simulink model "ReplayFlight_SensorMcu"  (Simulink 7.8)
settings: Solver=FixedStepDiscrete  StartTime=0.0  StopTime=time(end)  FixedStep=.01  RelTol=1e-3
values from neighbouring files (symbols this model uses):
  apSampleTime = 0.01    [Load_Replay.m]    (also in loadReplayMay2013.m; loadTuneRollReplay_May2013.m)
  baseHeight = GS_location(1)    [Load_Replay.m]    (also in loadReplayMay2013.m; loadTuneRollReplay_May2013.m)
  baseTemp = 288.215    [GetBaroAlt.m]
  GS_location = [180 36.9898376464844 -122.051963806152]    [Load_Replay.m]    (also in loadReplayMay2013.m; loadTuneRollReplay_May2013.m)
undefined symbols (not defined in the file or in its folder): barAdjust, baroCutTemp, baroOffset, baroScale, barTGain1, barTGain2, barTMean1, barTMean2, cubeAccelGain16405, cubeGyroGain16405, cubeMagGain16405, DiscIntNeverNeededParam, gaind, getGSLocation, Init_onlyOnce, Init_Reset, lapseRate, lowRateSensorCutoff, magMeanTemp, magOffset, magScale, magTempK, mainSensorCutoff, maxDynPressure, param_mag, pitAdjust, pitCutTemp, pitotOffset, pitotScale, pitTGain1, pitTGain2, pitTMean1, pitTMean2, polesd, powerOffset, powerScale, pressureSensorCutoff, q_quat, T, tempOffset, tempScale, Vb_0, y1, zerosd
libraries: aerolibconvert2 x10, simulink x7, SLUGS_Library x6, aerolibutil x4, dsPICdrivers x2, dspmtrx3 x1
(part 1 of 3)
settings Model: Creator=Administrator  LastModifiedBy=User
settings OptimizationCC: InitFltsAndDblsToZero=on
settings DebuggingCC: SaveWithParameterizedLinksMsg=none  FcnCallInpInsideContextMsg=Use local settings  StrictBusMsg=Warning
settings SFSimCC: SimParseCustomCode=off
settings GRTTargetCC: TargetFcnLib=ansi_tfl_tmw.mat

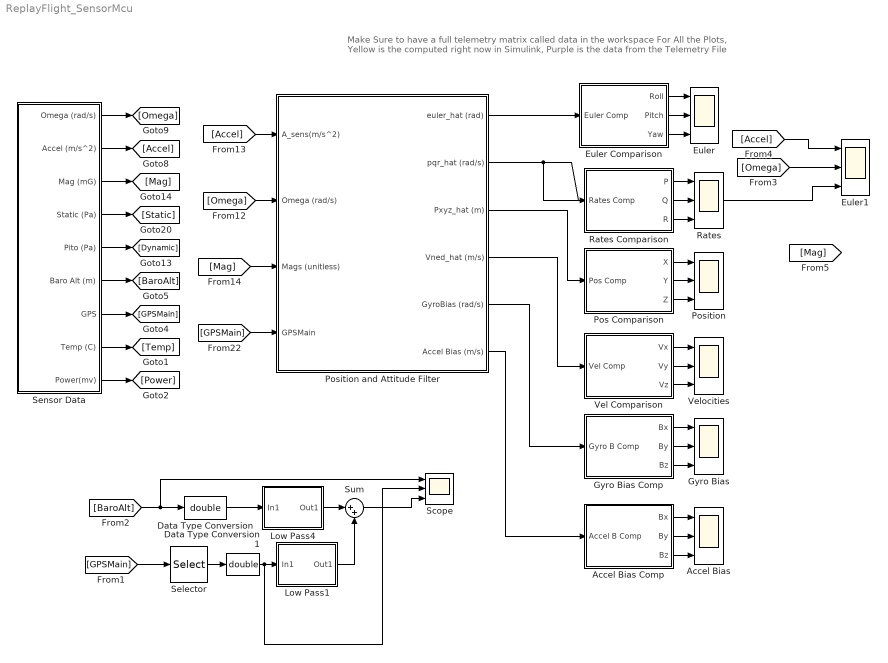
== system ReplayFlight_SensorMcu ==
  note: Make Sure to have a full telemetry matrix
      | called data in the workspace
      |
      | For All the Plots, Yellow is the computed right now in Simulink,
      |  Purple is the data from the Telemetry File
  Accel Bias : Scope  NumInputPorts=3
      settings: YMin=-5~-5~-5  YMax=5~5~5  SaveName=ScopeData5
  Accel Bias Comp : Subsystem
  Data Type Conversion : DataTypeConversion  OutDataTypeStr=double
  Data Type Conversion1 : DataTypeConversion  OutDataTypeStr=double
  Euler : Scope  NumInputPorts=3
      settings: YMin=-5~-5~-5  YMax=5~5~5
  Euler Comparison : Subsystem
  Euler1 : Scope  NumInputPorts=3
      settings: YMin=-5~-5~-5  YMax=5~5~5  SaveName=ScopeData7
  Gyro Bias : Scope  NumInputPorts=3
      settings: YMin=-5~-5~-5  YMax=5~5~5  SaveName=ScopeData4
  Gyro Bias Comp : Subsystem
  Low Pass1 : Subsystem  mask(DiscretizedZeroPole){Zeros=[0], Poles=[-1], Gain=1, AbsTol=auto, SampleTime=T, method=tustin, Wc=1}
      mask prompts: Zeros "Zeros (enter in s-main:)"; Poles "Poles (enter in s-domain:)"; Gain "Gain (enter in s-domain:)"; AbsTol "Absolute tolerance:"; SampleTime "Sample time:"; Wc "Critical Frequency (Hz):"
      mask help: Continuous mask uses c2d to transform parameters onto the Discrete Zero-Pole block inside.
      mask init:
      | st=SampleTime;
      | if length(st)>1
      |     st=SampleTime(1);
      | end
      | if(st>0)
      |     [zerosd,polesd,gaind] = sldiscutil('disczpk', {st,method,Wc,Zeros,Poles,Gain});
      | end	
      | s = get_param(gcb,'maskvalues');
      | zeross = s{1};
      | poless = s{2};
      | gainss = s{3};
      | %zerosc = eval(zeross);
      | %polesc = eval(poless);
      | %gainsc = eval(gainss);
      | sldiscutil('initzpkmask', st);
      | if(st==0)
      | set_param([gcb '/Zero Pole'], 'AbsoluteTolerance', AbsTol);
      | end
      mask StyleString: edit,edit,edit,edit,edit,popup(zoh|foh|tustin|prewarp|matched),edit
      mask CallbackString: |||||hidecrit|
      mask Display:
      | droots(zeross,poless,gainss)
      | text( 0.5, 1.0, method, 'verticalAlignment','top')
  Low Pass4 : Subsystem  mask(DiscretizedZeroPole){Zeros=[], Poles=[-0.3], Gain=0.3, AbsTol=auto, SampleTime=T, method=tustin, Wc=1}
      mask prompts: Zeros "Zeros (enter in s-main:)"; Poles "Poles (enter in s-domain:)"; Gain "Gain (enter in s-domain:)"; AbsTol "Absolute tolerance:"; SampleTime "Sample time:"; Wc "Critical Frequency (Hz):"
      mask help: Continuous mask uses c2d to transform parameters onto the Discrete Zero-Pole block inside.
      mask init: same as ReplayFlight_SensorMcu/Low Pass1
      mask StyleString: edit,edit,edit,edit,edit,popup(zoh|foh|tustin|prewarp|matched),edit
      mask CallbackString: |||||hidecrit|
      mask Display:
      | droots(zeross,poless,gainss)
      | text( 0.5, 1.0, method, 'verticalAlignment','top')
  Pos Comparison : Subsystem
  Position : Scope  NumInputPorts=3
      settings: YMin=-5~-5~-5  YMax=5~5~5  SaveName=ScopeData2
  Position and Attitude Filter : Subsystem
  Rates : Scope  NumInputPorts=3
      settings: YMin=-5~-5~-5  YMax=5~5~5
  Rates Comparison : Subsystem
  Scope : Scope  NumInputPorts=3
      settings: TimeRange=600  YMin=165.625~140~202.34375  YMax=386.875~280~333.59375  SaveName=ScopeData6
  Selector : Selector  InputPortWidth=5  IndexOptions=Index vector (dialog)  Indices=[3]  OutputSizes=1
  Sensor Data : Subsystem
  Sum : Sum  Inputs=|++
  Vel Comparison : Subsystem
  Velocities : Scope  NumInputPorts=3
      settings: YMin=-5~-5~-5  YMax=5~5~5  SaveName=ScopeData3
  wires:
  [Omega] -> Position and Attitude Filter/2(Omega (rad/s))
  [Accel] -> Position and Attitude Filter/1(A_sens(m/s^2))
  [Mag] -> Position and Attitude Filter/3(Mags (unitless))
  [GPSMain] -> Position and Attitude Filter/4(GPSMain)
  Sensor Data/2(Accel (m/s^2)) -> [Accel]
  Sensor Data/1(Omega (rad/s)) -> [Omega]
  Sensor Data/3(Mag (mG)) -> [Mag]
  Sensor Data/4(Static (Pa)) -> [Static]
  Sensor Data/5(Pito (Pa)) -> [Dynamic]
  Sensor Data/6(Baro Alt (m)) -> [BaroAlt]
  Sensor Data/7(GPS) -> [GPSMain]
  Sensor Data/8(Temp (C)) -> [Temp]
  Sensor Data/9(Power(mv)) -> [Power]
  Euler Comparison/1(Roll) -> Euler/1
  Euler Comparison/2(Pitch) -> Euler/2
  Euler Comparison/3(Yaw) -> Euler/3
  Position and Attitude Filter/1(euler_hat (rad)) -> Euler Comparison/1(Euler Comp)
  Rates Comparison/1(P) -> Rates/1
  Rates Comparison/2(Q) -> Rates/2
  Rates Comparison/3(R) -> Rates/3
  Position and Attitude Filter/2(pqr_hat (rad/s)) -> Rates Comparison/1(Rates Comp), Euler1/3
  Pos Comparison/3(Z) -> Position/3
  Position and Attitude Filter/3(Pxyz_hat (m)) -> Pos Comparison/1(Pos Comp)
  Pos Comparison/1(X) -> Position/1
  Pos Comparison/2(Y) -> Position/2
  Vel Comparison/3(Vz) -> Velocities/3
  Vel Comparison/2(Vy) -> Velocities/2
  Vel Comparison/1(Vx) -> Velocities/1
  Position and Attitude Filter/4(Vned_hat (m/s)) -> Vel Comparison/1(Vel Comp)
  Gyro Bias Comp/3(Bz) -> Gyro Bias/3
  Gyro Bias Comp/2(By) -> Gyro Bias/2
  Gyro Bias Comp/1(Bx) -> Gyro Bias/1
  Position and Attitude Filter/5(GyroBias (rad/s)) -> Gyro Bias Comp/1(Gyro B Comp)
  Accel Bias Comp/3(Bz) -> Accel Bias/3
  Accel Bias Comp/1(Bx) -> Accel Bias/1
  Accel Bias Comp/2(By) -> Accel Bias/2
  Position and Attitude Filter/6(Accel Bias (m/s)) -> Accel Bias Comp/1(Accel B Comp)
  [GPSMain] -> Selector/1
  [BaroAlt] -> Data Type Conversion/1, Scope/1
  Selector/1 -> Data Type Conversion1/1
  Low Pass4/1(Out1) -> Sum/1
  Low Pass1/1(Out1) -> Sum/2
  Sum/1 -> Scope/3
  Data Type Conversion/1 -> Low Pass4/1(In1)
  Data Type Conversion1/1 -> Low Pass1/1(In1), Scope/2
  [Omega] -> Euler1/2
  [Accel] -> Euler1/1

== system ReplayFlight_SensorMcu/Accel Bias Comp ==
  Accel B Comp : Inport
  Accel Bias : Subsystem
  Demux : Demux  Outputs=3
  Demux1 : Demux  Outputs=3
  Mux : Mux  Inputs=2
  Mux1 : Mux  Inputs=2
  Mux2 : Mux  Inputs=2
  Bx : Outport
  By : Outport  Port=2
  Bz : Outport  Port=3
  wires:
  Demux1/3 -> Mux2/2
  Demux1/2 -> Mux1/2
  Demux1/1 -> Mux/2
  Accel Bias/1(A bias) -> Demux1/1
  Demux/3 -> Mux2/1
  Demux/2 -> Mux1/1
  Demux/1 -> Mux/1
  Accel B Comp/1 -> Demux/1
  Mux2/1 -> Bz/1
  Mux1/1 -> By/1
  Mux/1 -> Bx/1

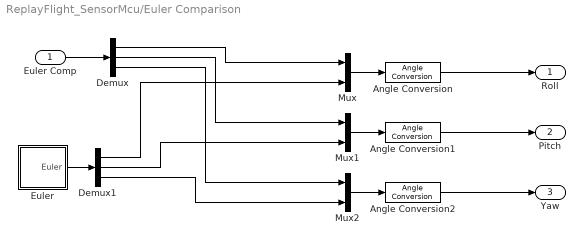
== system ReplayFlight_SensorMcu/Euler Comparison ==
  Euler Comp : Inport
  Angle Conversion : aerolibconvert2/Angle Conversion  IU=rad  OU=deg
  Angle Conversion1 : aerolibconvert2/Angle Conversion  IU=rad  OU=deg
  Angle Conversion2 : aerolibconvert2/Angle Conversion  IU=rad  OU=deg
  Demux : Demux  Outputs=3
  Demux1 : Demux  Outputs=3
  Euler : Subsystem
  Mux : Mux  Inputs=2
  Mux1 : Mux  Inputs=2
  Mux2 : Mux  Inputs=2
  Roll : Outport
  Pitch : Outport  Port=2
  Yaw : Outport  Port=3
  wires:
  Mux/1 -> Angle Conversion/1
  Mux1/1 -> Angle Conversion1/1
  Mux2/1 -> Angle Conversion2/1
  Euler Comp/1 -> Demux/1
  Demux/1 -> Mux/1
  Demux/2 -> Mux1/1
  Demux/3 -> Mux2/1
  Euler/1(Euler) -> Demux1/1
  Demux1/1 -> Mux/2
  Demux1/2 -> Mux1/2
  Demux1/3 -> Mux2/2
  Angle Conversion/1 -> Roll/1
  Angle Conversion1/1 -> Pitch/1
  Angle Conversion2/1 -> Yaw/1

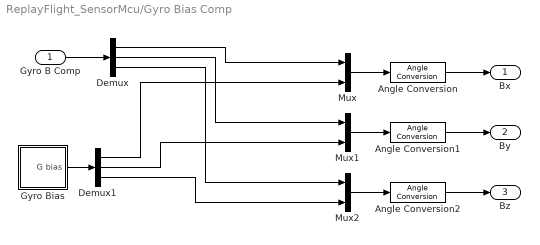
== system ReplayFlight_SensorMcu/Gyro Bias Comp ==
  Gyro B Comp : Inport
  Angle Conversion : aerolibconvert2/Angle Conversion  IU=rad  OU=deg
  Angle Conversion1 : aerolibconvert2/Angle Conversion  IU=rad  OU=deg
  Angle Conversion2 : aerolibconvert2/Angle Conversion  IU=rad  OU=deg
  Demux : Demux  Outputs=3
  Demux1 : Demux  Outputs=3
  Gyro Bias : Subsystem
  Mux : Mux  Inputs=2
  Mux1 : Mux  Inputs=2
  Mux2 : Mux  Inputs=2
  Bx : Outport
  By : Outport  Port=2
  Bz : Outport  Port=3
  wires:
  Mux/1 -> Angle Conversion/1
  Mux1/1 -> Angle Conversion1/1
  Mux2/1 -> Angle Conversion2/1
  Gyro B Comp/1 -> Demux/1
  Demux/1 -> Mux/1
  Demux/2 -> Mux1/1
  Demux/3 -> Mux2/1
  Gyro Bias/1(G bias) -> Demux1/1
  Demux1/1 -> Mux/2
  Demux1/2 -> Mux1/2
  Demux1/3 -> Mux2/2
  Angle Conversion/1 -> Bx/1
  Angle Conversion1/1 -> By/1
  Angle Conversion2/1 -> Bz/1

== system ReplayFlight_SensorMcu/Low Pass1 ==
  In1 : Inport
  Discrete Zero-Pole : DiscreteZeroPole  Zeros=zerosd  Poles=polesd  Gain=gaind  SampleTime=SampleTime
  Out1 : Outport
  wires:
  Discrete Zero-Pole/1 -> Out1/1
  In1/1 -> Discrete Zero-Pole/1

== system ReplayFlight_SensorMcu/Low Pass4 ==
  In1 : Inport
  Discrete Zero-Pole : DiscreteZeroPole  Zeros=zerosd  Poles=polesd  Gain=gaind  SampleTime=SampleTime
  Out1 : Outport
  wires:
  In1/1 -> Discrete Zero-Pole/1
  Discrete Zero-Pole/1 -> Out1/1

== system ReplayFlight_SensorMcu/Pos Comparison ==
  Pos Comp : Inport
  Demux : Demux  Outputs=3
  Demux1 : Demux  Outputs=3
  Mux : Mux  Inputs=2
  Mux1 : Mux  Inputs=2
  Mux2 : Mux  Inputs=2
  Pos : Subsystem
  X : Outport
  Y : Outport  Port=2
  Z : Outport  Port=3
  wires:
  Mux/1 -> X/1
  Mux1/1 -> Y/1
  Mux2/1 -> Z/1
  Pos Comp/1 -> Demux/1
  Demux/1 -> Mux/1
  Demux/2 -> Mux1/1
  Demux/3 -> Mux2/1
  ? -> Demux1/1
  Demux1/1 -> Mux/2
  Demux1/2 -> Mux1/2
  Demux1/3 -> Mux2/2

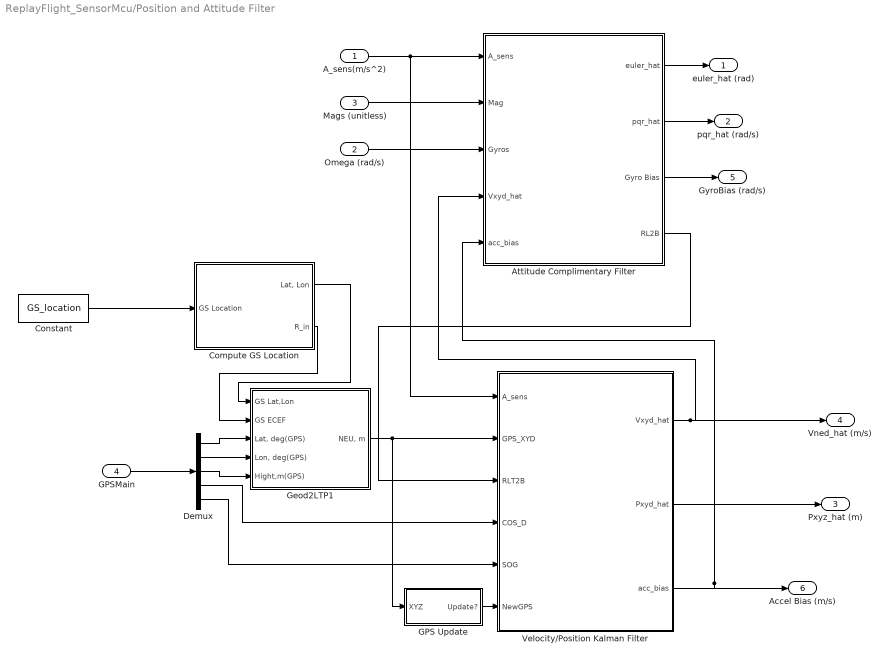
== system ReplayFlight_SensorMcu/Position and Attitude Filter ==
  A_sens(m/s^2) : Inport
  Omega (rad/s) : Inport  Port=2
  Mags (unitless) : Inport  Port=3
  GPSMain : Inport  Port=4
  Attitude Complimentary Filter : Subsystem
  Compute GS Location : Subsystem
  Constant : Constant  Value=GS_location  OutDataTypeStr=single
  Demux : Demux  Outputs=5
  GPS Update : Subsystem  mask{T=0.01}
      mask prompts: T "Sample Time"
  Geod2LTP1 : Subsystem
      mask Description:
      | This block provides transformation of the Geodetic coordinates
      | to the LTP coorinate system. The block uses two consecutive transformations
      | (Geodetic -> ECEF ->LTP).
      | Geodetic coordinates of the LTP origin should also be predetermined.
      mask Help: Oops!
      mask Display: plot(0,0,100,100,[45,40,35,40,40],[85,95,85,95,40],[85,95,85,95,40],[35,40,45,40,40],[60,40,10,20,10,14],[70,40,10,13,10,20],[56,45],[70,70],[60,60],[50,60],[60,60],[30,40],[50,60],[20,20],[30,40],[20,20],[45,55],[35,25],[75,65],[35,25])
  Velocity/Position Kalman Filter : MATLAB Function  TreatAsAtomicUnit=on
  euler_hat (rad) : Outport
  pqr_hat (rad/s) : Outport  Port=2
  Pxyz_hat (m) : Outport  Port=3
  Vned_hat (m/s) : Outport  Port=4
  GyroBias (rad/s) : Outport  Port=5
  Accel Bias (m/s) : Outport  Port=6
  wires:
  Omega (rad/s)/1 -> Attitude Complimentary Filter/3(Gyros)
  Mags (unitless)/1 -> Attitude Complimentary Filter/2(Mag)
  A_sens(m/s^2)/1 -> Attitude Complimentary Filter/1(A_sens), Velocity/Position Kalman Filter/1(A_sens)
  GPS Update/1(Update?) -> Velocity/Position Kalman Filter/6(NewGPS)
  Compute GS Location/1("Lat, Lon") -> Geod2LTP1/1(GS Lat,Lon)
  Compute GS Location/2(R_in) -> Geod2LTP1/2(GS ECEF)
  Demux/3 -> Geod2LTP1/5(Hight,m(GPS))
  Demux/2 -> Geod2LTP1/4("Lon, deg(GPS)")
  Demux/1 -> Geod2LTP1/3("Lat, deg(GPS)")
  Constant/1 -> Compute GS Location/1(GS Location)
  Demux/5 -> Velocity/Position Kalman Filter/5(SOG)
  Demux/4 -> Velocity/Position Kalman Filter/4(COS_D)
  GPSMain/1 -> Demux/1
  Attitude Complimentary Filter/3(Gyro Bias) -> GyroBias (rad/s)/1
  Attitude Complimentary Filter/2(pqr_hat) -> pqr_hat (rad/s)/1
  Attitude Complimentary Filter/1(euler_hat) -> euler_hat (rad)/1
  Attitude Complimentary Filter/4(RL2B) -> Velocity/Position Kalman Filter/3(RLT2B)
  Geod2LTP1/1("NEU, m") -> Velocity/Position Kalman Filter/2(GPS_XYD), GPS Update/1(XYZ)
  Velocity/Position Kalman Filter/3(acc_bias) -> Accel Bias (m/s)/1, Attitude Complimentary Filter/5(acc_bias)
  Velocity/Position Kalman Filter/2(Pxyd_hat) -> Pxyz_hat (m)/1
  Velocity/Position Kalman Filter/1(Vxyd_hat) -> Vned_hat (m/s)/1, Attitude Complimentary Filter/4(Vxyd_hat)

== system ReplayFlight_SensorMcu/Rates Comparison ==
  Rates Comp : Inport
  Angle Conversion : aerolibconvert2/Angle Conversion  IU=rad  OU=deg
  Angle Conversion1 : aerolibconvert2/Angle Conversion  IU=rad  OU=deg
  Angle Conversion2 : aerolibconvert2/Angle Conversion  IU=rad  OU=deg
  Demux : Demux  Outputs=3
  Demux1 : Demux  Outputs=3
  Mux : Mux  Inputs=2
  Mux1 : Mux  Inputs=2
  Mux2 : Mux  Inputs=2
  Rates : Subsystem
  P : Outport
  Q : Outport  Port=2
  R : Outport  Port=3
  wires:
  Angle Conversion2/1 -> R/1
  Angle Conversion1/1 -> Q/1
  Angle Conversion/1 -> P/1
  Demux1/3 -> Mux2/2
  Demux1/2 -> Mux1/2
  Demux1/1 -> Mux/2
  Rates/1(Rates) -> Demux1/1
  Demux/3 -> Mux2/1
  Demux/2 -> Mux1/1
  Demux/1 -> Mux/1
  Rates Comp/1 -> Demux/1
  Mux2/1 -> Angle Conversion2/1
  Mux1/1 -> Angle Conversion1/1
  Mux/1 -> Angle Conversion/1

== system ReplayFlight_SensorMcu/Sensor Data ==
  Sensor Suite : Subsystem
  Omega (rad/s) : Outport
  Accel (m/s^2) : Outport  Port=2
  Mag (mG) : Outport  Port=3
  Static (Pa) : Outport  Port=4
  Pito (Pa) : Outport  Port=5
  Baro Alt (m) : Outport  Port=6
  GPS : Outport  Port=7
  Temp (C) : Outport  Port=8
  Power(mv) : Outport  Port=9
  wires:
  Sensor Suite/7(GPS) -> GPS/1
  Sensor Suite/6(Baro Alt (m)) -> Baro Alt (m)/1
  Sensor Suite/5(Pitot (Pa)) -> Pito (Pa)/1
  Sensor Suite/4(Static (Pa)) -> Static (Pa)/1
  Sensor Suite/3(Mag (normalized)) -> Mag (mG)/1
  Sensor Suite/2(Accel (m/s^2)) -> Accel (m/s^2)/1
  Sensor Suite/1(Omega (rad/s)) -> Omega (rad/s)/1
  Sensor Suite/8(Temp(C)) -> Temp (C)/1
  Sensor Suite/9(Power) -> Power(mv)/1

== system ReplayFlight_SensorMcu/Vel Comparison ==
  Vel Comp : Inport
  Demux : Demux  Outputs=3
  Demux1 : Demux  Outputs=3
  Mux : Mux  Inputs=2
  Mux1 : Mux  Inputs=2
  Mux2 : Mux  Inputs=2
  Vel : Subsystem
  Vx : Outport
  Vy : Outport  Port=2
  Vz : Outport  Port=3
  wires:
  Demux1/3 -> Mux2/2
  Demux1/2 -> Mux1/2
  Demux1/1 -> Mux/2
  ? -> Demux1/1
  Demux/3 -> Mux2/1
  Demux/2 -> Mux1/1
  Demux/1 -> Mux/1
  Vel Comp/1 -> Demux/1
  Mux2/1 -> Vz/1
  Mux1/1 -> Vy/1
  Mux/1 -> Vx/1

== system ReplayFlight_SensorMcu/Accel Bias Comp/Accel Bias ==
  Data Type Conversion3 : DataTypeConversion  OutDataTypeStr=single
  Mux : Mux  Inputs=3
  p : FromWorkspace  VariableName=[time ABI_comp(:,1)]  SampleTime=0.01  OutputAfterFinalValue=Setting to zero
  p1 : FromWorkspace  VariableName=[time ABI_comp(:,2)]  SampleTime=0.01  OutputAfterFinalValue=Setting to zero
  p2 : FromWorkspace  VariableName=[time ABI_comp(:,3)]  SampleTime=0.01  OutputAfterFinalValue=Setting to zero
  A bias : Outport
  wires:
  Data Type Conversion3/1 -> A bias/1
  Mux/1 -> Data Type Conversion3/1
  p2/1 -> Mux/3
  p1/1 -> Mux/2
  p/1 -> Mux/1

== system ReplayFlight_SensorMcu/Euler Comparison/Euler ==
  Data Type Conversion3 : DataTypeConversion  OutDataTypeStr=single
  Mux : Mux  Inputs=3
  p : FromWorkspace  VariableName=[time EUL_comp(:,1)]  SampleTime=0.01  OutputAfterFinalValue=Setting to zero
  p1 : FromWorkspace  VariableName=[time EUL_comp(:,2)]  SampleTime=0.01  OutputAfterFinalValue=Setting to zero
  p2 : FromWorkspace  VariableName=[time EUL_comp(:,3)]  SampleTime=0.01  OutputAfterFinalValue=Setting to zero
  Euler : Outport
  wires:
  p/1 -> Mux/1
  p1/1 -> Mux/2
  p2/1 -> Mux/3
  Mux/1 -> Data Type Conversion3/1
  Data Type Conversion3/1 -> Euler/1

== system ReplayFlight_SensorMcu/Gyro Bias Comp/Gyro Bias ==
  Data Type Conversion3 : DataTypeConversion  OutDataTypeStr=single
  Mux : Mux  Inputs=3
  p : FromWorkspace  VariableName=[time GBI_comp(:,1)]  SampleTime=0.01  OutputAfterFinalValue=Setting to zero
  p1 : FromWorkspace  VariableName=[time GBI_comp(:,2)]  SampleTime=0.01  OutputAfterFinalValue=Setting to zero
  p2 : FromWorkspace  VariableName=[time GBI_comp(:,3)]  SampleTime=0.01  OutputAfterFinalValue=Setting to zero
  G bias : Outport
  wires:
  p/1 -> Mux/1
  p1/1 -> Mux/2
  p2/1 -> Mux/3
  Mux/1 -> Data Type Conversion3/1
  Data Type Conversion3/1 -> G bias/1

== system ReplayFlight_SensorMcu/Pos Comparison/Pos ==
  Data Type Conversion3 : DataTypeConversion  OutDataTypeStr=single
  Mux : Mux  Inputs=3
  p : FromWorkspace  VariableName=[time POS_comp(:,1)]  SampleTime=0.01  OutputAfterFinalValue=Setting to zero
  p1 : FromWorkspace  VariableName=[time POS_comp(:,2)]  SampleTime=0.01  OutputAfterFinalValue=Setting to zero
  p2 : FromWorkspace  VariableName=[time POS_comp(:,3)]  SampleTime=0.01  OutputAfterFinalValue=Setting to zero
  Position : Outport
  wires:
  p/1 -> Mux/1
  p1/1 -> Mux/2
  p2/1 -> Mux/3
  Mux/1 -> Data Type Conversion3/1
  Data Type Conversion3/1 -> Position/1

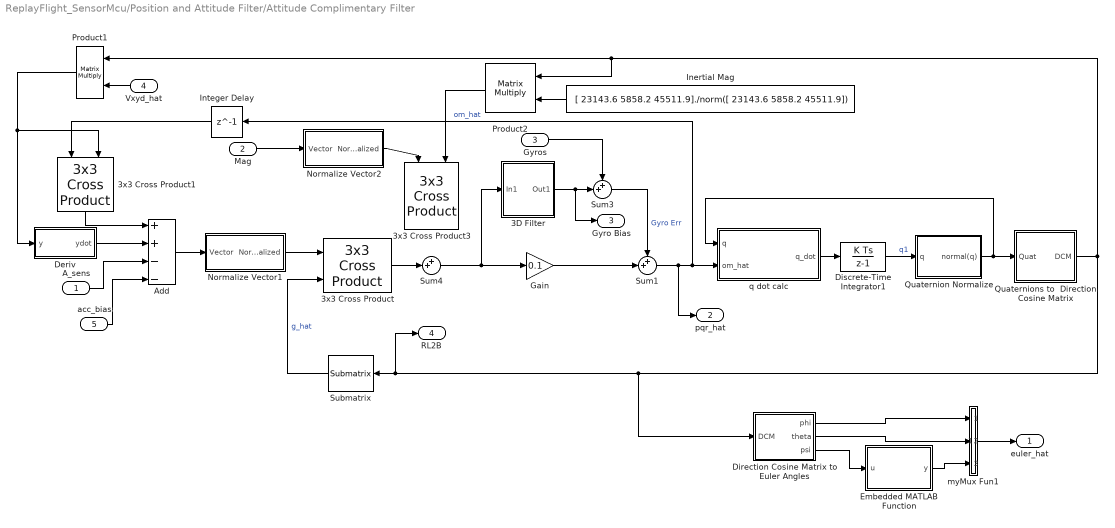
== system ReplayFlight_SensorMcu/Position and Attitude Filter/Attitude Complimentary Filter ==
  A_sens : Inport  PortDimensions=3
  Mag : Inport  Port=2  PortDimensions=3
  Gyros : Inport  Port=3  PortDimensions=3
  Vxyd_hat : Inport  Port=4  PortDimensions=3
  acc_bias : Inport  Port=5  PortDimensions=3
  3D Filter : Subsystem  AncestorBlock=SLUGS_Library/Singnal Routing & Conditioning/3D Filter  RTWFcnName=TustinFilter3D  mask{zval=[], pval=[0], kval=.003, TSample=0.01}
      mask prompts: zval "Zeros"; pval "Poles"; kval "Gains"; TSample "Sample Time"
      settings: RTWFcnNameOpts=User specified  RTWFileNameOpts=Use function name
      mask Display:
      | droots(zval,pval,kval)
      | port_label('input',1,'3D')
  3x3 Cross Product : aerolibutil/3x3 Cross Product
  3x3 Cross Product1 : aerolibutil/3x3 Cross Product
  3x3 Cross Product3 : aerolibutil/3x3 Cross Product
  Add : Sum  Inputs=++--
  "Deriv " : Subsystem
  Direction Cosine Matrix to Euler Angles : Subsystem  AncestorBlock=aerolibtransform2/Direction Cosine Matrix to Euler Angles  mask(DCM2Euler){}
      mask help: Determine an euler orientation (roll, pitch, yaw) from the 3-by-3 direction cosine matrix (DCM). The input DCM transforms vectors from geodetic earth or north-down-east (NED) axes to body axes.
      mask init:
      | aeroicon('aeroblk');
      mask Help: web(asbhelp('directioncosinematrixtoeulerangles'));
      mask Display:
      | port_label('output',1,'\phi','texmode','on')
      | port_label('output',2,'\theta','texmode','on')
      | port_label('output',3,'\psi','texmode','on')
      | port_label('input',1,'DCM_{be}','texmode','on')
  Discrete-Time Integrator1 : DiscreteIntegrator  InitialCondition=q_quat  SampleTime=apSampleTime  LimitOutput=on  UpperSaturationLimit=[1 1 1 1]  LowerSaturationLimit=[-1 -1 -1 -1]  ICPrevOutput=DiscIntNeverNeededParam  ICPrevScaledInput=DiscIntNeverNeededParam
  Embedded MATLAB Function : MATLAB Function  TreatAsAtomicUnit=on
  Gain : Gain  Gain=0.1
  Inertial Mag : Constant  Value="[ 23143.6   5858.2    45511.9]./norm([ 23143.6   5858.2    45511.9])"  OutDataTypeStr=single
  Integer Delay : Delay  DelayLength=1  InputProcessing=Inherited
  Normalize Vector1 : Subsystem  AncestorBlock=SLUGS_Library/Navigation/Normalize Vector
  Normalize Vector2 : Subsystem  AncestorBlock=SLUGS_Library/Navigation/Normalize Vector
  Product1 : Product  Multiplication=Matrix(*)  RndMeth=Zero
  Product2 : Product  Multiplication=Matrix(*)  RndMeth=Zero
  Quaternion Normalize : Subsystem  AncestorBlock=aerolibutil/Quaternion Normalize  mask(Quaternion Normalize){}
      mask help: Normalize a quaternion.
      mask init:
      | aeroicon('aeroblk');
      mask Help: web(asbhelp);
  Quaternions to  Direction Cosine Matrix : Subsystem  AncestorBlock="aerolibtransform2/Quaternions to  Direction Cosine Matrix"  mask(Quaternion2DCM){}
      mask help: Determine the 3-by-3 direction cosine matrix (DCM) from a 4-by-1 quaternion orientation vector. The output DCM transforms vectors from geodetic earth or north-east-down (NED) axes to body axes.
      mask init:
      | aeroicon('aeroblk');
      mask Help: web(asbhelp('quaternionstodirectioncosinematrix'));
      mask Display:
      | port_label('input',1,'q_n_o_r_m','texmode','on')
      | port_label('output',1,'DCM_{be}','texmode','on')
  Submatrix : dspmtrx3/Submatrix  RowSpan=Range of rows  RowStartMode=First  RowStartIndex=1  RowEndMode=Last  RowEndIndex=1  ColSpan=One column  ColStartMode=Last  ColStartIndex=1  ColEndMode=Last  ColEndIndex=1
  Sum1 : Sum  Inputs=++|
  Sum3 : Sum  Inputs=++|
  Sum4 : Sum  Inputs=++|
  myMux Fun1 : MATLAB Function  TreatAsAtomicUnit=on
  q dot calc : MATLAB Function  TreatAsAtomicUnit=on
  euler_hat : Outport
  pqr_hat : Outport  Port=2
  Gyro Bias : Outport  Port=3
  RL2B : Outport  Port=4
  wires:
  Normalize Vector2/1(Normalized) -> 3x3 Cross Product3/1
  Sum3/1 -> Sum1/1  "Gyro Err"
  Gain/1 -> Sum1/2
  Gyros/1 -> Sum3/1
  3D Filter/1(Out1) -> Sum3/2, Gyro Bias/1
  Embedded MATLAB Function/1(y) -> myMux Fun1/3(u3)
  Direction Cosine Matrix to Euler Angles/2(theta) -> myMux Fun1/2(u2)
  Direction Cosine Matrix to Euler Angles/1(phi) -> myMux Fun1/1(u1)
  myMux Fun1/1(y) -> euler_hat/1
  Direction Cosine Matrix to Euler Angles/3(psi) -> Embedded MATLAB Function/1(u)
  Vxyd_hat/1 -> Product1/2
  Product1/1 -> "Deriv "/1(y), 3x3 Cross Product1/2
  Mag/1 -> Normalize Vector2/1(Vector)
  acc_bias/1 -> Add/4
  Add/1 -> Normalize Vector1/1(Vector)
  "Deriv "/1(ydot) -> Add/2
  Quaternion Normalize/1(normal(q)) -> q dot calc/1(q), Quaternions to  Direction Cosine Matrix/1(Quat)
  Discrete-Time Integrator1/1 -> Quaternion Normalize/1(q)  "q1"
  Integer Delay/1 -> 3x3 Cross Product1/1
  Inertial Mag/1 -> Product2/2
  Quaternions to  Direction Cosine Matrix/1(DCM) -> Direction Cosine Matrix to Euler Angles/1(DCM), RL2B/1, Submatrix/1, Product1/1, Product2/1
  Product2/1 -> 3x3 Cross Product3/2
  3x3 Cross Product/1 -> Sum4/2
  Normalize Vector1/1(Normalized) -> 3x3 Cross Product/1
  A_sens/1 -> Add/3
  3x3 Cross Product1/1 -> Add/1
  Sum4/1 -> 3D Filter/1(In1), Gain/1
  Submatrix/1 -> 3x3 Cross Product/2  "g_hat"
  q dot calc/1(q_dot) -> Discrete-Time Integrator1/1
  Sum1/1 -> pqr_hat/1, Integer Delay/1, q dot calc/2(om_hat)  "om_hat"

== system ReplayFlight_SensorMcu/Position and Attitude Filter/Compute GS Location ==
  GS Location : Inport
  Demux : Demux  Outputs=3
  Geod2ECEF1 : Subsystem  mask{Re=6378137, Rp=6356752.3142}
      mask prompts: Re "Enter equatorial radius, m"; Rp "Enter polar radius,m"
  Mux1 : Mux  Inputs=2
  Mux2 : Mux  Inputs=3
  "Lat, Lon" : Outport
  R_in : Outport  Port=2
  wires:
  Mux2/1 -> R_in/1  "R_in"
  Mux1/1 -> "Lat, Lon"/1
  GS Location/1 -> Demux/1
  Demux/3 -> Geod2ECEF1/3(lon,deg), Mux1/1
  Demux/2 -> Geod2ECEF1/2("lat, deg"), Mux1/2
  Demux/1 -> Geod2ECEF1/1("height, m")
  Geod2ECEF1/2("Ye, m ") -> Mux2/2
  Geod2ECEF1/1("Xe, m ") -> Mux2/1
  Geod2ECEF1/3("Ze, m ") -> Mux2/3

== system ReplayFlight_SensorMcu/Position and Attitude Filter/GPS Update ==
  XYZ : Inport
  Data Type Conversion2 : DataTypeConversion  OutDataTypeStr=uint8
  Demux : Demux  Outputs=3
  Detect Change : Subsystem
  Detect Change1 : Subsystem
  Detect Change2 : Subsystem
  Rate Transition : RateTransition  OutPortSampleTime=T
  Saturation1 : Saturate  UpperLimit=1  LowerLimit=0  SampleTime=T
  Sum : Sum  Inputs=3
  Update? : Outport
  wires:
  Data Type Conversion2/1 -> Update?/1
  Rate Transition/1 -> Demux/1
  Saturation1/1 -> Data Type Conversion2/1
  XYZ/1 -> Rate Transition/1
  Sum/1 -> Saturation1/1
  Detect Change2/1(change?) -> Sum/3
  Detect Change1/1(change?) -> Sum/2
  Detect Change/1(change?) -> Sum/1
  Demux/3 -> Detect Change2/1(Data)
  Demux/2 -> Detect Change1/1(Data)
  Demux/1 -> Detect Change/1(Data)

== system ReplayFlight_SensorMcu/Position and Attitude Filter/Geod2LTP1 ==
  GS Lat,Lon : Inport
  GS ECEF : Inport  Port=2
  "Lat, deg(GPS)" : Inport  Port=3
  "Lon, deg(GPS)" : Inport  Port=4
  Hight,m(GPS) : Inport  Port=5
  ECEF2LTP (UEN) : Subsystem
      mask Display: plot(0,0,100,100,[45,40,35,40,40],[85,95,85,95,40],[85,95,85,95,40],[35,40,45,40,40],[60,40,10,20,10,14],[70,40,10,13,10,20],[56,45],[70,70],[60,60],[50,60],[60,60],[30,40],[50,60],[20,20],[30,40],[20,20],[45,55],[35,25],[75,65],[35,25])
  Geod2ECEF1 : Subsystem  mask{Re=6378137, Rp=6356752.3142}
      mask prompts: Re "Enter equatorial radius, m"; Rp "Enter polar radius,m"
  Mux : Mux  Inputs=3
  Reshape : Reshape  OutputDimensionality=Column vector (2-D)
  Reshape1 : Reshape
  Sum1 : Sum  Inputs=|+-  OutDataTypeStr=single  SaturateOnIntegerOverflow=on
  UEN 2 NEU : Gain  Gain=[0 0 1;0 1 0;1 0 0]  Multiplication=Matrix(K*u)  OutDataTypeStr=float('single')  SaturateOnIntegerOverflow=on  ParamDataTypeStr=Inherit: Same as input
  "NEU, m" : Outport
  wires:
  UEN 2 NEU/1 -> Reshape1/1
  Geod2ECEF1/3("Ze, m ") -> Mux/3
  Geod2ECEF1/1("Xe, m ") -> Mux/1
  Geod2ECEF1/2("Ye, m ") -> Mux/2
  "Lat, deg(GPS)"/1 -> Geod2ECEF1/2("lat, deg")
  "Lon, deg(GPS)"/1 -> Geod2ECEF1/3(lon,deg)
  GS Lat,Lon/1 -> ECEF2LTP (UEN)/2("Long, Lat")
  GS ECEF/1 -> Sum1/2
  ECEF2LTP (UEN)/1(Out) -> Reshape/1  "Moving Side"
  Hight,m(GPS)/1 -> Geod2ECEF1/1("height, m")
  Mux/1 -> Sum1/1  "r_mov"
  Sum1/1 -> ECEF2LTP (UEN)/1(ECEF coordinates)
  Reshape/1 -> UEN 2 NEU/1
  Reshape1/1 -> "NEU, m"/1

== system ReplayFlight_SensorMcu/Rates Comparison/Rates ==
  Data Type Conversion3 : DataTypeConversion  OutDataTypeStr=single
  Mux : Mux  Inputs=3
  p : FromWorkspace  VariableName=[time PQR_comp(:,1)]  SampleTime=0.01  OutputAfterFinalValue=Setting to zero
  p1 : FromWorkspace  VariableName=[time PQR_comp(:,2)]  SampleTime=0.01  OutputAfterFinalValue=Setting to zero
  p2 : FromWorkspace  VariableName=[time PQR_comp(:,3)]  SampleTime=0.01  OutputAfterFinalValue=Setting to zero
  Rates : Outport
  wires:
  Data Type Conversion3/1 -> Rates/1
  Mux/1 -> Data Type Conversion3/1
  p2/1 -> Mux/3
  p1/1 -> Mux/2
  p/1 -> Mux/1

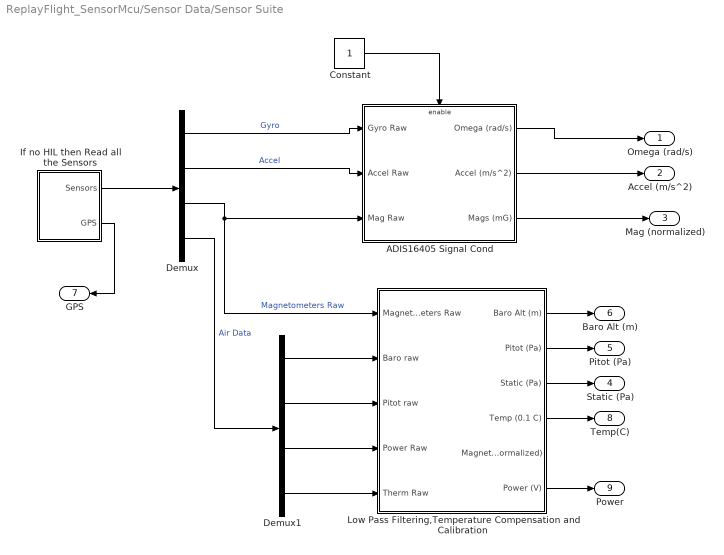
== system ReplayFlight_SensorMcu/Sensor Data/Sensor Suite ==
  "ADIS16405 Signal Cond " : Subsystem
  Constant : Constant
  Demux : Demux  Outputs=[3 3 3 4]
  Demux1 : Demux
  If no HIL then Read all the Sensors : Subsystem
  Low Pass Filtering,Temperature Compensation and Calibration : Subsystem
  Omega (rad/s) : Outport
  Accel (m/s^2) : Outport  Port=2
  Mag (normalized) : Outport  Port=3
  Static (Pa) : Outport  Port=4
  Pitot (Pa) : Outport  Port=5
  Baro Alt (m) : Outport  Port=6
  GPS : Outport  Port=7
  Temp(C) : Outport  Port=8
  Power : Outport  Port=9
  wires:
  Demux/2 -> "ADIS16405 Signal Cond "/2(Accel Raw)  "Accel"
  Low Pass Filtering,Temperature Compensation and Calibration/3(Static (Pa)) -> Static (Pa)/1
  Low Pass Filtering,Temperature Compensation and Calibration/2(Pitot (Pa)) -> Pitot (Pa)/1
  Demux1/3 -> Low Pass Filtering,Temperature Compensation and Calibration/4(Power Raw)
  Demux/3 -> Low Pass Filtering,Temperature Compensation and Calibration/1(Magnetometers Raw), "ADIS16405 Signal Cond "/3(Mag Raw)  "Magnetometers Raw"
  Demux1/4 -> Low Pass Filtering,Temperature Compensation and Calibration/5(Therm Raw)
  Demux1/2 -> Low Pass Filtering,Temperature Compensation and Calibration/3(Pitot raw)
  Demux1/1 -> Low Pass Filtering,Temperature Compensation and Calibration/2(Baro raw)
  Demux/4 -> Demux1/1  "Air Data"
  Demux/1 -> "ADIS16405 Signal Cond "/1(Gyro Raw)  "Gyro"
  Low Pass Filtering,Temperature Compensation and Calibration/1(Baro Alt (m)) -> Baro Alt (m)/1
  If no HIL then Read all the Sensors/1(Sensors) -> Demux/1
  If no HIL then Read all the Sensors/2(GPS) -> GPS/1
  Low Pass Filtering,Temperature Compensation and Calibration/6(Power (V)) -> Power/1
  Low Pass Filtering,Temperature Compensation and Calibration/4(Temp (0.1 C)) -> Temp(C)/1
  "ADIS16405 Signal Cond "/1(Omega (rad/s)) -> Omega (rad/s)/1
  "ADIS16405 Signal Cond "/2(Accel (m/s^2)) -> Accel (m/s^2)/1
  "ADIS16405 Signal Cond "/3(Mags (mG)) -> Mag (normalized)/1
  Constant/1 -> "ADIS16405 Signal Cond "/Enable

== system ReplayFlight_SensorMcu/Vel Comparison/Vel ==
  Data Type Conversion3 : DataTypeConversion  OutDataTypeStr=single
  Mux : Mux  Inputs=3
  p : FromWorkspace  VariableName=[time VEL_comp(:,1)]  SampleTime=0.01  OutputAfterFinalValue=Setting to zero
  p1 : FromWorkspace  VariableName=[time VEL_comp(:,2)]  SampleTime=0.01  OutputAfterFinalValue=Setting to zero
  p2 : FromWorkspace  VariableName=[time VEL_comp(:,3)]  SampleTime=0.01  OutputAfterFinalValue=Setting to zero
  Vel : Outport
  wires:
  Data Type Conversion3/1 -> Vel/1
  Mux/1 -> Data Type Conversion3/1
  p2/1 -> Mux/3
  p1/1 -> Mux/2
  p/1 -> Mux/1

== system ReplayFlight_SensorMcu/Position and Attitude Filter/Attitude Complimentary Filter/3D Filter ==
  In1 : Inport
  Data Type Conversion1 : DataTypeConversion  OutDataTypeStr=single
  Data Type Conversion2 : DataTypeConversion  OutDataTypeStr=double
  Demux : Demux  Outputs=3
  Filter1 : Subsystem  mask(DiscretizedZeroPole){Zeros=zval, Poles=pval, Gain=kval, AbsTol=auto, SampleTime=TSample, method=tustin, Wc=1}
      mask prompts: Zeros "Zeros (enter in s-main:)"; Poles "Poles (enter in s-domain:)"; Gain "Gain (enter in s-domain:)"; AbsTol "Absolute tolerance:"; SampleTime "Sample time:"; Wc "Critical Frequency (Hz):"
      mask help: Continuous mask uses c2d to transform parameters onto the Discrete Zero-Pole block inside.
      mask init: same as ReplayFlight_SensorMcu/Low Pass1
      mask StyleString: edit,edit,edit,edit,edit,popup(zoh|foh|tustin|prewarp|matched),edit
      mask CallbackString: |||||hidecrit|
      mask Display:
      | droots(zeross,poless,gainss)
      | text( 0.5, 1.0, method, 'verticalAlignment','top')
  Filter2 : Subsystem  mask(DiscretizedZeroPole){Zeros=zval, Poles=pval, Gain=kval, AbsTol=auto, SampleTime=TSample, method=tustin, Wc=1}
      mask prompts: Zeros "Zeros (enter in s-main:)"; Poles "Poles (enter in s-domain:)"; Gain "Gain (enter in s-domain:)"; AbsTol "Absolute tolerance:"; SampleTime "Sample time:"; Wc "Critical Frequency (Hz):"
      mask help: Continuous mask uses c2d to transform parameters onto the Discrete Zero-Pole block inside.
      mask init: same as ReplayFlight_SensorMcu/Low Pass1
      mask StyleString: edit,edit,edit,edit,edit,popup(zoh|foh|tustin|prewarp|matched),edit
      mask CallbackString: |||||hidecrit|
      mask Display:
      | droots(zeross,poless,gainss)
      | text( 0.5, 1.0, method, 'verticalAlignment','top')
  Filter3 : Subsystem  mask(DiscretizedZeroPole){Zeros=zval, Poles=pval, Gain=kval, AbsTol=auto, SampleTime=TSample, method=tustin, Wc=1}
      mask prompts: Zeros "Zeros (enter in s-main:)"; Poles "Poles (enter in s-domain:)"; Gain "Gain (enter in s-domain:)"; AbsTol "Absolute tolerance:"; SampleTime "Sample time:"; Wc "Critical Frequency (Hz):"
      mask help: Continuous mask uses c2d to transform parameters onto the Discrete Zero-Pole block inside.
      mask init: same as ReplayFlight_SensorMcu/Low Pass1
      mask StyleString: edit,edit,edit,edit,edit,popup(zoh|foh|tustin|prewarp|matched),edit
      mask CallbackString: |||||hidecrit|
      mask Display:
      | droots(zeross,poless,gainss)
      | text( 0.5, 1.0, method, 'verticalAlignment','top')
  myMux Fun1 : MATLAB Function  TreatAsAtomicUnit=on
  Out1 : Outport
  wires:
  Data Type Conversion1/1 -> Out1/1
  Data Type Conversion2/1 -> Demux/1
  Demux/1 -> Filter1/1(In1)
  Demux/2 -> Filter2/1(In1)
  Demux/3 -> Filter3/1(In1)
  Filter1/1(Out1) -> myMux Fun1/1(u1)
  Filter2/1(Out1) -> myMux Fun1/2(u2)
  Filter3/1(Out1) -> myMux Fun1/3(u3)
  In1/1 -> Data Type Conversion2/1
  myMux Fun1/1(y) -> Data Type Conversion1/1

== system ReplayFlight_SensorMcu/Position and Attitude Filter/Attitude Complimentary Filter/Deriv  ==
  y : Inport
  Gain2 : Gain  Gain=[ 1/(5*apSampleTime) ]
  Integer Delay1 : Delay  DelayLength=5  InitialCondition=Vb_0(1)  InputProcessing=Inherited  SampleTime=apSampleTime
  Sum5 : Sum  Inputs=-+|
  ydot : Outport
  wires:
  Gain2/1 -> ydot/1
  y/1 -> Integer Delay1/1, Sum5/2
  Integer Delay1/1 -> Sum5/1
  Sum5/1 -> Gain2/1

== system ReplayFlight_SensorMcu/Position and Attitude Filter/Attitude Complimentary Filter/Direction Cosine Matrix to Euler Angles ==
  DCM : Inport  PortDimensions=[3,3]
  "Reshape 3x3 -> 9" : Reshape  OutputDimensions=[9, 1]
  Subsystem1 : SLUGS_Library/Subsystem4
  Subsystem2 : SLUGS_Library/Subsystem4
  Subsystem3 : SLUGS_Library/Subsystem6
  cos(phi)cos(theta) : Subsystem
  cos(psi)cos(theta) : Subsystem
  sin(phi)cos(theta) : Subsystem
  sin(psi)cos(theta) : Subsystem
  sin(theta) : Subsystem
  phi : Outport  PortDimensions=1  InitialOutput=0
  theta : Outport  Port=2  PortDimensions=1  InitialOutput=0
  psi : Outport  Port=3  PortDimensions=1  InitialOutput=0
  wires:
  Subsystem1/1 -> psi/1  "psi"
  Subsystem3/1 -> theta/1  "theta"
  Subsystem2/1 -> phi/1  "phi"
  cos(psi)cos(theta)/1(cos(psi)cos(theta)) -> Subsystem1/2
  sin(psi)cos(theta)/1(sin(psi)cos(theta)) -> Subsystem1/1
  cos(phi)cos(theta)/1(cos(phi)cos(theta)) -> Subsystem2/2
  sin(phi)cos(theta)/1(sin(phi)cos(theta)) -> Subsystem2/1
  sin(theta)/1(sin(theta)) -> Subsystem3/1
  "Reshape 3x3 -> 9"/1 -> sin(psi)cos(theta)/1(DCM), cos(psi)cos(theta)/1(DCM), sin(phi)cos(theta)/1(DCM), cos(phi)cos(theta)/1(DCM), sin(theta)/1(DCM)
  DCM/1 -> "Reshape 3x3 -> 9"/1

== system ReplayFlight_SensorMcu/Position and Attitude Filter/Attitude Complimentary Filter/Normalize Vector1 ==
  Vector : Inport
  Divide : Product  Inputs=*/
  Norm : Subsystem  AncestorBlock=SLUGS_Library/Navigation/Norm
  Zero Bound : Saturate  UpperLimit=inf  LowerLimit=0.001
  Normalized : Outport
  wires:
  Vector/1 -> Norm/1(Vector), Divide/1
  Norm/1(Norm) -> Zero Bound/1
  Zero Bound/1 -> Divide/2
  Divide/1 -> Normalized/1

== system ReplayFlight_SensorMcu/Position and Attitude Filter/Attitude Complimentary Filter/Normalize Vector2 ==
  Vector : Inport
  Divide : Product  Inputs=*/
  Norm : Subsystem  AncestorBlock=SLUGS_Library/Navigation/Norm
  Zero Bound : Saturate  UpperLimit=inf  LowerLimit=0.001
  Normalized : Outport
  wires:
  Divide/1 -> Normalized/1
  Zero Bound/1 -> Divide/2
  Norm/1(Norm) -> Zero Bound/1
  Vector/1 -> Divide/1, Norm/1(Vector)

== system ReplayFlight_SensorMcu/Position and Attitude Filter/Attitude Complimentary Filter/Quaternion Normalize ==
  q : Inport
  Demux : Demux
  Mux : Mux
  Product{,1..3} (4 alike) : Product  Inputs=*/
  Quaternion Modulus : Subsystem  AncestorBlock=aerolibutil/Quaternion Modulus  mask(Quaternion Modulus){}
      mask help: Calculate the modulus of a quaternion.
      mask init:
      | aeroicon('aeroblk');
      mask Help: web(asbhelp);
  normal(q) : Outport
  wires:
  Demux/4 -> Product3/1
  Demux/3 -> Product2/1
  Demux/2 -> Product1/1
  Demux/1 -> Product/1
  Mux/1 -> normal(q)/1
  q/1 -> Demux/1, Quaternion Modulus/1(q)
  Quaternion Modulus/1(|q|) -> Product1/2, Product/2, Product2/2, Product3/2
  Product/1 -> Mux/1
  Product1/1 -> Mux/2
  Product2/1 -> Mux/3
  Product3/1 -> Mux/4

== system ReplayFlight_SensorMcu/Position and Attitude Filter/Attitude Complimentary Filter/Quaternions to  Direction Cosine Matrix ==
  Quat : Inport  PortDimensions=4
  A11 : Subsystem
  A12 : Subsystem
  A13 : Subsystem
  A21 : Subsystem
  A22 : Subsystem
  A23 : Subsystem
  A31 : Subsystem
  A32 : Subsystem
  A33 : Subsystem
  Create Transformation Matrix : Subsystem  AncestorBlock=aerolibutil/Create 3x3 Matrix  mask(Create 3x3 Matrix){}
      mask help:
      | Create a 3-by-3 matrix from nine input values. Each input corresponds to an element of the matrix.
      |
      | For example, the input labeled A21 is the entry in the second row and first column of the matrix.
      mask init:
      | aeroicon('aeroblk');
      mask Help: web(asbhelp);
      mask Display:
      | port_label('input',1,'A_{11}','texmode','on');
      | port_label('input',2,'A_{12}','texmode','on');
      | port_label('input',3,'A_{13}','texmode','on');
      | port_label('input',4,'A_{21}','texmode','on');
      | port_label('input',5,'A_{22}','texmode','on');
      | port_label('input',6,'A_{23}','texmode','on');
      | port_label('input',7,'A_{31}','texmode','on');
      | port_label('input',8,'A_{32}','texmode','on');
      | port_label('input',9,'A_{33}','texmode','on');
      | port_label('output',1,'A','texmode','on');
  DCM : Outport  PortDimensions=[3,3]  InitialOutput=0
  wires:
  Create Transformation Matrix/1(Matrix) -> DCM/1
  A11/1(A11) -> Create Transformation Matrix/1(M11)
  A21/1(A21) -> Create Transformation Matrix/4(M21)
  A31/1(A31) -> Create Transformation Matrix/7(M31)
  A32/1(A32) -> Create Transformation Matrix/8(M32)
  A13/1(A13) -> Create Transformation Matrix/3(M13)
  A23/1(A23) -> Create Transformation Matrix/6(M23)
  A33/1(A33) -> Create Transformation Matrix/9(M33)
  Quat/1 -> A33/1(normal(q)), A32/1(normal(q)), A31/1(normal(q)), A23/1(normal(q)), A22/1(normal(q)), A21/1(normal(q)), A13/1(normal(q)), A12/1(normal(q)), A11/1(normal(q))
  A22/1(A22) -> Create Transformation Matrix/5(M22)
  A12/1(A12) -> Create Transformation Matrix/2(M12)

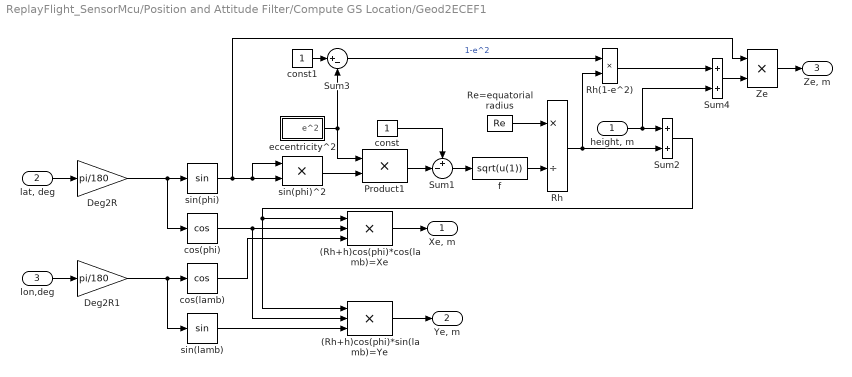
== system ReplayFlight_SensorMcu/Position and Attitude Filter/Compute GS Location/Geod2ECEF1 ==
  "height, m" : Inport
  "lat, deg" : Inport  Port=2
  lon,deg : Inport  Port=3
  (Rh+h)cos(phi)*cos(lamb)=Xe : Product  Inputs=3  OutDataTypeStr=single  SaturateOnIntegerOverflow=on  InputSameDT=on
  (Rh+h)cos(phi)*sin(lamb)=Ye : Product  Inputs=3  OutDataTypeStr=single  SaturateOnIntegerOverflow=on  InputSameDT=on
  Deg2R : Gain  Gain=pi/180  OutDataTypeStr=float('single')  SaturateOnIntegerOverflow=on  ParamDataTypeStr=Inherit: Same as input
  Deg2R1 : Gain  Gain=pi/180  OutDataTypeStr=float('single')  SaturateOnIntegerOverflow=on  ParamDataTypeStr=Inherit: Same as input
  Product1 : Product  SaturateOnIntegerOverflow=on  InputSameDT=on  OutDataTypeStr=Inherit: Same as first input
  Re=equatorial radius : Constant  Value=Re  OutDataTypeStr=single
  Rh : Product  Inputs=*/  OutDataTypeStr=single  SaturateOnIntegerOverflow=on  InputSameDT=on
  Rh(1-e^2) : Product  OutDataTypeStr=single  SaturateOnIntegerOverflow=on  InputSameDT=on
  Sum1 : Sum  Inputs=+-|  SaturateOnIntegerOverflow=on  InputSameDT=on  OutDataTypeStr=Inherit: Same as first input
  Sum2 : Sum  SaturateOnIntegerOverflow=on  InputSameDT=on  OutDataTypeStr=Inherit: Same as first input
      settings: AttributesFormatString=Rh+h
  Sum3 : Sum  Inputs=|+-  SaturateOnIntegerOverflow=on  InputSameDT=on  OutDataTypeStr=Inherit: Same as first input
  Sum4 : Sum  OutDataTypeStr=single  SaturateOnIntegerOverflow=on  InputSameDT=on
      settings: AttributesFormatString=(1-e^2)Rh+h
  Ze : Product  OutDataTypeStr=single  SaturateOnIntegerOverflow=on  InputSameDT=on
  const : Constant  OutDataTypeStr=single
  const1 : Constant  OutDataTypeStr=single
  cos(lamb) : Trigonometry  Operator=cos
  cos(phi) : Trigonometry  Operator=cos
  eccentricity^2 : Subsystem
  f : Fcn  Expr=sqrt(u(1))
  sin(lamb) : Trigonometry
  sin(phi) : Trigonometry
  sin(phi)^2 : Product  SaturateOnIntegerOverflow=on  InputSameDT=on  OutDataTypeStr=Inherit: Same as first input
  "Xe, m " : Outport
  "Ye, m " : Outport  Port=2
  "Ze, m " : Outport  Port=3
  wires:
  "lat, deg"/1 -> Deg2R/1
  sin(phi)/1 -> sin(phi)^2/1, sin(phi)^2/2, Ze/1
  f/1 -> Rh/2
  Re=equatorial radius/1 -> Rh/1
  Rh/1 -> Sum2/2, Rh(1-e^2)/2
  Product1/1 -> Sum1/2
  Sum1/1 -> f/1
  const/1 -> Sum1/1
  "height, m"/1 -> Sum4/2, Sum2/1
  eccentricity^2/1(e^2) -> Product1/1, Sum3/2
  sin(phi)^2/1 -> Product1/2
  const1/1 -> Sum3/1
  Sum3/1 -> Rh(1-e^2)/1  "1-e^2"
  Rh(1-e^2)/1 -> Sum4/1
  Sum4/1 -> Ze/2
  lon,deg/1 -> Deg2R1/1
  cos(phi)/1 -> (Rh+h)cos(phi)*cos(lamb)=Xe/2, (Rh+h)cos(phi)*sin(lamb)=Ye/2
  cos(lamb)/1 -> (Rh+h)cos(phi)*cos(lamb)=Xe/3
  sin(lamb)/1 -> (Rh+h)cos(phi)*sin(lamb)=Ye/3
  Ze/1 -> "Ze, m "/1
  Deg2R/1 -> cos(phi)/1, sin(phi)/1
  Deg2R1/1 -> cos(lamb)/1, sin(lamb)/1
  Sum2/1 -> (Rh+h)cos(phi)*sin(lamb)=Ye/1, (Rh+h)cos(phi)*cos(lamb)=Xe/1
  (Rh+h)cos(phi)*cos(lamb)=Xe/1 -> "Xe, m "/1
  (Rh+h)cos(phi)*sin(lamb)=Ye/1 -> "Ye, m "/1

== system ReplayFlight_SensorMcu/Position and Attitude Filter/GPS Update/Detect Change ==
  Data : Inport
  Abs1 : Abs  SampleTime=T
  Difference1 : simulink/Discrete/Difference  ICPrevInput=0.0  InputProcessing=Inherited  OutMin=[]  OutMax=[]  OutDataType=sfix(16)  OutScaling=2^-10  DoSatur=off
  Saturation1 : Saturate  UpperLimit=1  LowerLimit=0  SampleTime=T
  change? : Outport
  wires:
  Saturation1/1 -> change?/1
  Data/1 -> Difference1/1
  Abs1/1 -> Saturation1/1
  Difference1/1 -> Abs1/1

== system ReplayFlight_SensorMcu/Position and Attitude Filter/GPS Update/Detect Change1 ==
  Data : Inport
  Abs1 : Abs  SampleTime=T
  Difference1 : simulink/Discrete/Difference  ICPrevInput=0.0  InputProcessing=Inherited  OutMin=[]  OutMax=[]  OutDataType=sfix(16)  OutScaling=2^-10  DoSatur=off
  Saturation1 : Saturate  UpperLimit=1  LowerLimit=0  SampleTime=T
  change? : Outport
  wires:
  Difference1/1 -> Abs1/1
  Abs1/1 -> Saturation1/1
  Data/1 -> Difference1/1
  Saturation1/1 -> change?/1

== system ReplayFlight_SensorMcu/Position and Attitude Filter/GPS Update/Detect Change2 ==
  Data : Inport
  Abs1 : Abs  SampleTime=T
  Difference1 : simulink/Discrete/Difference  ICPrevInput=0.0  InputProcessing=Inherited  OutMin=[]  OutMax=[]  OutDataType=sfix(16)  OutScaling=2^-10  DoSatur=off
  Saturation1 : Saturate  UpperLimit=1  LowerLimit=0  SampleTime=T
  change? : Outport
  wires:
  Saturation1/1 -> change?/1
  Data/1 -> Difference1/1
  Abs1/1 -> Saturation1/1
  Difference1/1 -> Abs1/1

== system ReplayFlight_SensorMcu/Position and Attitude Filter/Geod2LTP1/ECEF2LTP (UEN) ==
  ECEF coordinates : Inport
  "Long, Lat" : Inport  Port=2
  Deg2R : Gain  Gain=pi/180  SaturateOnIntegerOverflow=on  OutDataTypeStr=Inherit: Same as input  ParamDataTypeStr=Inherit: Same as input
  Demux3 : Demux  Outputs=2
  From Body to Universal1 : Subsystem
  Product1 : Product  Multiplication=Matrix(*)  SaturateOnIntegerOverflow=on  InputSameDT=on  OutDataTypeStr=Inherit: Same as first input
  Out : Outport
  wires:
  "Long, Lat"/1 -> Deg2R/1
  Product1/1 -> Out/1
  Demux3/2 -> From Body to Universal1/2(lat)
  Demux3/1 -> From Body to Universal1/1(long)
  Deg2R/1 -> Demux3/1
  ECEF coordinates/1 -> Product1/2
  From Body to Universal1/1(DCM) -> Product1/1

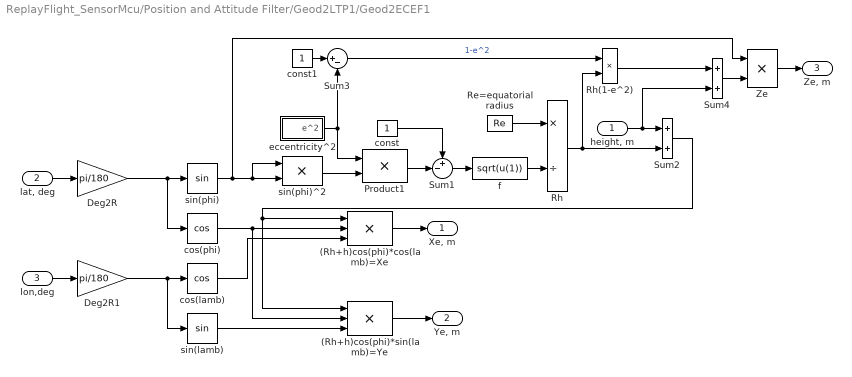
== system ReplayFlight_SensorMcu/Position and Attitude Filter/Geod2LTP1/Geod2ECEF1 ==
  "height, m" : Inport
  "lat, deg" : Inport  Port=2
  lon,deg : Inport  Port=3
  (Rh+h)cos(phi)*cos(lamb)=Xe : Product  Inputs=3  OutDataTypeStr=single  SaturateOnIntegerOverflow=on  InputSameDT=on
  (Rh+h)cos(phi)*sin(lamb)=Ye : Product  Inputs=3  OutDataTypeStr=single  SaturateOnIntegerOverflow=on  InputSameDT=on
  Deg2R : Gain  Gain=pi/180  OutDataTypeStr=float('single')  SaturateOnIntegerOverflow=on  ParamDataTypeStr=Inherit: Same as input
  Deg2R1 : Gain  Gain=pi/180  OutDataTypeStr=float('single')  SaturateOnIntegerOverflow=on  ParamDataTypeStr=Inherit: Same as input
  Product1 : Product  SaturateOnIntegerOverflow=on  InputSameDT=on  OutDataTypeStr=Inherit: Same as first input
  Re=equatorial radius : Constant  Value=Re  OutDataTypeStr=single
  Rh : Product  Inputs=*/  OutDataTypeStr=single  SaturateOnIntegerOverflow=on  InputSameDT=on
  Rh(1-e^2) : Product  OutDataTypeStr=single  SaturateOnIntegerOverflow=on  InputSameDT=on
  Sum1 : Sum  Inputs=+-|  SaturateOnIntegerOverflow=on  InputSameDT=on  OutDataTypeStr=Inherit: Same as first input
  Sum2 : Sum  SaturateOnIntegerOverflow=on  InputSameDT=on  OutDataTypeStr=Inherit: Same as first input
      settings: AttributesFormatString=Rh+h
  Sum3 : Sum  Inputs=|+-  SaturateOnIntegerOverflow=on  InputSameDT=on  OutDataTypeStr=Inherit: Same as first input
  Sum4 : Sum  OutDataTypeStr=single  SaturateOnIntegerOverflow=on  InputSameDT=on
      settings: AttributesFormatString=(1-e^2)Rh+h
  Ze : Product  OutDataTypeStr=single  SaturateOnIntegerOverflow=on  InputSameDT=on
  const : Constant  OutDataTypeStr=single
  const1 : Constant  OutDataTypeStr=single
  cos(lamb) : Trigonometry  Operator=cos
  cos(phi) : Trigonometry  Operator=cos
  eccentricity^2 : Subsystem
  f : Fcn  Expr=sqrt(u(1))
  sin(lamb) : Trigonometry
  sin(phi) : Trigonometry
  sin(phi)^2 : Product  SaturateOnIntegerOverflow=on  InputSameDT=on  OutDataTypeStr=Inherit: Same as first input
  "Xe, m " : Outport
  "Ye, m " : Outport  Port=2
  "Ze, m " : Outport  Port=3
  wires:
  "lat, deg"/1 -> Deg2R/1
  sin(phi)/1 -> sin(phi)^2/1, sin(phi)^2/2, Ze/1
  f/1 -> Rh/2
  Re=equatorial radius/1 -> Rh/1
  Rh/1 -> Sum2/2, Rh(1-e^2)/2
  Product1/1 -> Sum1/2
  Sum1/1 -> f/1
  const/1 -> Sum1/1
  "height, m"/1 -> Sum4/2, Sum2/1
  eccentricity^2/1(e^2) -> Product1/1, Sum3/2
  sin(phi)^2/1 -> Product1/2
  const1/1 -> Sum3/1
  Sum3/1 -> Rh(1-e^2)/1  "1-e^2"
  Rh(1-e^2)/1 -> Sum4/1
  Sum4/1 -> Ze/2
  lon,deg/1 -> Deg2R1/1
  cos(phi)/1 -> (Rh+h)cos(phi)*cos(lamb)=Xe/2, (Rh+h)cos(phi)*sin(lamb)=Ye/2
  cos(lamb)/1 -> (Rh+h)cos(phi)*cos(lamb)=Xe/3
  sin(lamb)/1 -> (Rh+h)cos(phi)*sin(lamb)=Ye/3
  Ze/1 -> "Ze, m "/1
  Deg2R/1 -> cos(phi)/1, sin(phi)/1
  Deg2R1/1 -> cos(lamb)/1, sin(lamb)/1
  Sum2/1 -> (Rh+h)cos(phi)*sin(lamb)=Ye/1, (Rh+h)cos(phi)*cos(lamb)=Xe/1
  (Rh+h)cos(phi)*cos(lamb)=Xe/1 -> "Xe, m "/1
  (Rh+h)cos(phi)*sin(lamb)=Ye/1 -> "Ye, m "/1
